simulink model "DNNCells_tSPMeA_BatteryPack_Passive100cellBal_RestCycler"  (R2024a)
settings: Solver=VariableStepAuto  StartTime=0.0  StopTime=1E7  RelTol=1e-3
undefined symbols (not defined in the file or in its folder): battery_builder_rtmsupport, gcbh
libraries: fl_lib x38, nesl_utility x36, simulink x26, BatteryLibrary_lib x6
(part 1 of 2)
settings Model: LastModifiedBy=Carlos

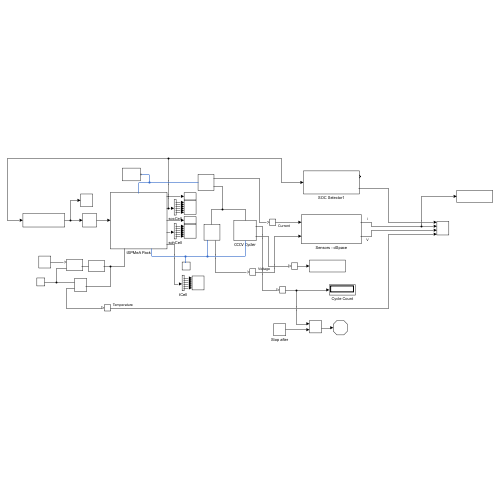
[thumbnail: Simulink's stored preview of the top-level diagram]
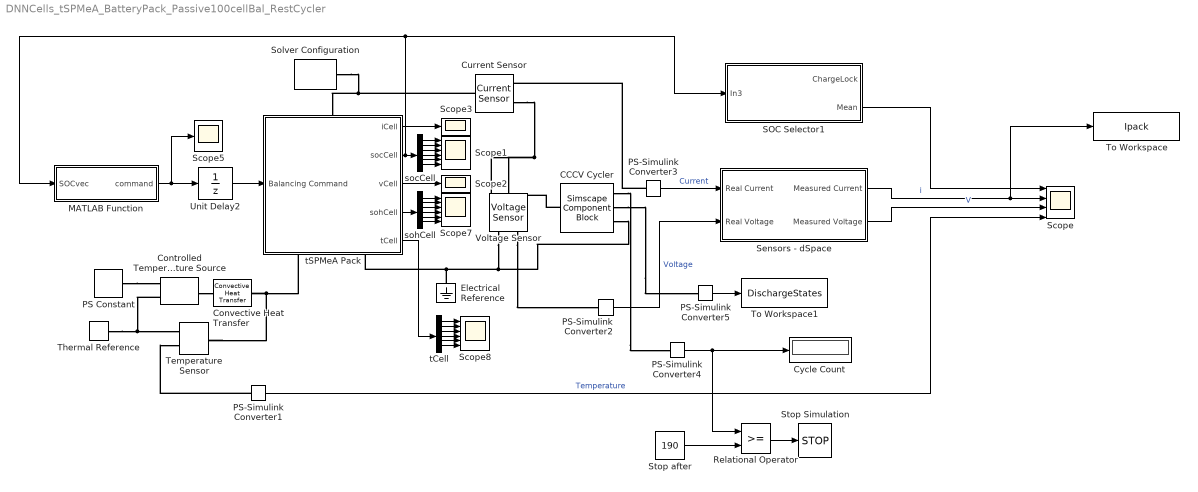
== system DNNCells_tSPMeA_BatteryPack_Passive100cellBal_RestCycler ==
  CCCV Cycler : SimscapeComponentBlock  SourceFile=BatteryCycler_CCCV_DischargeInd  ComponentPath=BatteryCycler_CCCV_DischargeInd  ComponentVariants="[\"BatteryCycler_CCCV_DischargeInd\"]"  ComponentVariantNames="[\"BatteryCycler_CCCV_DischargeInd\"]"  ClassName=BatteryCycler_CCCV_DischargeInd  SchemaVersion=1  Vmax=12.2 V  Vmin=minV V  Ic=iValueC A  Ico=0.25*3 A  Id=iValueD A  tRestC=0 s  tRestD=0 s
      settings: CopyFcn=simscape.engine.sli.internal.componentblockcallback(gcbh,'COPY')  PreCopyFcn=simscape.engine.sli.internal.componentblockcallback(gcbh,'PRECOPY')  PreDeleteFcn=simscape.engine.sli.internal.componentblockcallback(gcbh,'PREDELETE')  InternalSimscapePortConfiguration="{\"Bottom\":[{\"id\":\"n\",\"label\":\"-\",\"type\":\"foundation.electrical.electrical\"}],\"Left\":[],\"Right\":[{\"id\":\"numCyc\",\"label\":\"Cyc#\",\"type\":\"output\"},{\"id\":\"DischargeON\",\"label\":\"dON\",\"type\":\"output\"}],\"Top\":[{\"id\":\"p\",\"label\":\"+\",\"type\":\"foundation.electrical.electrical\"}]}"
      mask Type: A simple battery cycler
      mask Display: color('red');plot([0 1 1 0 0],[0 0 1 1 0]);plot([0.7,1],[1,0.7]);plot(-2,-1.75);plot(3, 1);disp('\n.ssc\nUnresolved')
  Controlled Temperature Source : fl_lib/Thermal/Thermal Sources/Controlled Temperature Source
  Convective Heat Transfer : fl_lib/Thermal/Thermal Elements/Convective Heat Transfer  thermal_type=foundation.enum.constant_variable.constant  area=0.1019 m^2  heat_tr_coeff=5 W/(K*m^2)  min_heat_tr_coeff=1e-3 W/(K*m^2)  T_specify=off  T_priority=None  T=0 K  T_nominal_specify=off  T_nominal_value=1  T_nominal_unit=K  Q_specify=off  Q_priority=None  Q=0 W  Q_nominal_specify=off  Q_nominal_value=1  Q_nominal_unit=W
  Current Sensor : fl_lib/Electrical/Electrical Sensors/Current Sensor
  Cycle Count : Display
  Electrical Reference : fl_lib/Electrical/Electrical Elements/Electrical Reference
  MATLAB Function : MATLAB Function  TreatAsAtomicUnit=on
  PS Constant : fl_lib/Physical Signals/Sources/PS Constant  constant=Rtemp K
  PS-Simulink Converter{1..5} (5 alike) : nesl_utility/PS-Simulink Converter  PhysicalDomain=network_engine_domain  SubClassName=ps_output  LeftPortType=input  RightPortType=output  PseudoPeriodic=off  Frequencies=[]  VectorFormat=inherit  Unit=inherit  AffineConversion=off
  Relational Operator : RelationalOperator  OutDataTypeStr=boolean  RndMeth=Simplest  InputSameDT=off
  SOC Selector1 : Subsystem
  Scope : Scope  NumInputPorts=4
  Scope1 : Scope  NumInputPorts=6
  Scope2 : Scope
  Scope3 : Scope
  Scope5 : Scope
  Scope7 : Scope  NumInputPorts=6
  Scope8 : Scope  NumInputPorts=6
  Sensors - dSpace : Subsystem
  Solver Configuration : nesl_utility/Solver Configuration  PhysicalDomain=network_engine_domain  SubClassName=solver  LeftPortType=input  RightPortType=generic  Tones=[]  Harmonics=[]  SimulateNoise=off  Profile=off  UseLocalSampling=off  EnableSwitchedLinearOptims=on  FrequencyDomain=off  UseCCode=off  RelTol=0.001  AbsTol=0.001  MinStep=1e-09  ToWorkspace=off  RevertToSquareIcSolve=off  NumHomotopyIterations=100  PhasorMode=off  PhasorModeNumHarmonics=1  ConsistencySolver=NEWTON_XTOL_AFTER_FTOL  IndexReductionMethod=DerivativeReplacement  DoDC=off  ResidualTolerance=1e-09  ConsistencyTolSource=GLOBAL  ConsistencyAbsTol=0.001  ConsistencyRelTol=0.001  ConsistencyTolFactor=0.001  UseLocalSolver=off  LocalSolverChoice=NE_BACKWARD_EULER_ADVANCER  ResolveIndetEquations=on  FunctionEvalNumThread=1  LocalSolverSampleTime=0.001  DoFixedCost=off  MaxNonlinIter=3  MaxModeIter=2  ComputeImpulses=off  ImpulseIterations=2  LinearAlgebra=auto  LinearAlgebraNumThread=0  EquationFormulation=NE_TIME_EF  DelaysMemoryBudget=1024  AutomaticFiltering=on  FilteringTimeConstant=0.001  PartitionStorageMethod=AS_NEEDED  PartitionMemoryBudget=1024  PartitionMethod=ROBUST  MultibodyUseLocalSolver=off  MultibodyLocalSolverChoice=ODE1  MultibodyLocalSolverSampleTime=0.001
  Stop Simulation : Stop
  Stop after : Constant  Value=190
  Temperature Sensor : fl_lib/Thermal/Thermal Sensors/Temperature Sensor  temperature_measure=foundation.enum.MeasurementReference.difference
  Thermal Reference : fl_lib/Thermal/Thermal Elements/Thermal Reference
  To Workspace : ToWorkspace  VariableName=Ipack  SampleTime=-1
  To Workspace1 : ToWorkspace  VariableName=DischargeStates  SampleTime=-1
  Unit Delay2 : UnitDelay  SampleTime=-1  HasFrameUpgradeWarning=on
  Voltage Sensor : fl_lib/Electrical/Electrical Sensors/Voltage Sensor
  socCell : Demux  Outputs=6
  sohCell : Demux  Outputs=6
  tCell : Demux  Outputs=6
  tSPMeA Pack : Subsystem  LoadFcn=battery_builder_rtmsupport('loadfcn',gcbh);
      settings: CopyFcn=battery_builder_rtmsupport('copyfcn',gcbh);  PreCopyFcn=battery_builder_rtmsupport('precopyfcn',gcbh);  PreDeleteFcn=battery_builder_rtmsupport('predeletefcn',gcbh);  PortSchema="{\"entries\":[{\"content\":{\"sides\":[{\"content\":{\"connectorIds\":[\"LConn1\"]},\"type\":\"ConnectorPlacement.EquallySpacedRectSide\",\"uuid\":\"edb5d46f-daf4-45ed-b1d9-08af295e59c6\"},{\"content\":{\"connectorIds\":[\"RConn1\",\"RConn2\"],\"side\":\"RIGHT\"},\"type\":\"ConnectorPlacement.EquallySpacedRectSide\",\"uuid\":\"7cebd990-2869-4bd2-9528-842d68f5845c\"},{\"content\":{\"connectorIds\":[\"In1\"],\"side\":\"TOP\"},\"type\":\"ConnectorPlacement.EquallySpacedRectSide\",\"uuid\":\"ba73c8cc-44ad-460a-9725-00030624eda5\"},{\"content\":{\"connectorIds\":[\"Out1\",\"Out2\",\"Out3\",\"Out4\",\"Out5\"],\"side\":\"BOTTOM\"},\"type\":\"ConnectorPlacement.EquallySpacedRectSide\",\"uuid\":\"cf00b7fe-9012-41be-869c-9f0653cf4178\"}]},\"type\":\"ConnectorPlacement.EquallySpacedConnector\",\"uuid\":\"85879143-d5a0-4157-9373-c0baeacbbffb\"}],\"packageUris\":[\"http://schema.mathworks.com/mf0/Connector/R2020b\"],\"version\":\"1.0\"}"
      mask Display: image('$imagefile')
  wires:
  tSPMeA Pack/2(socCell) -> socCell/1, MATLAB Function/1(SOCvec), SOC Selector1/1(In3)
  PS-Simulink Converter1/1 -> Scope/4  "Temperature"
  tSPMeA Pack/1(iCell) -> Scope3/1
  socCell/1 -> Scope1/1
  PS-Simulink Converter2/1 -> Sensors - dSpace/2(Real Voltage)  "Voltage"
  Sensors - dSpace/1(Measured Current) -> To Workspace/1, Scope/2  "i"
  Sensors - dSpace/2(Measured Voltage) -> Scope/3  "V"
  socCell/2 -> Scope1/2
  socCell/3 -> Scope1/3
  socCell/4 -> Scope1/4
  socCell/5 -> Scope1/5
  socCell/6 -> Scope1/6
  Unit Delay2/1 -> tSPMeA Pack/1(Balancing Command)
  tSPMeA Pack/3(vCell) -> Scope2/1
  MATLAB Function/1(command) -> Scope5/1, Unit Delay2/1
  tSPMeA Pack/4(sohCell) -> sohCell/1
  sohCell/1 -> Scope7/1
  sohCell/2 -> Scope7/2
  sohCell/3 -> Scope7/3
  sohCell/4 -> Scope7/4
  sohCell/5 -> Scope7/5
  sohCell/6 -> Scope7/6
  tCell/5 -> Scope8/5
  tCell/1 -> Scope8/1
  tCell/6 -> Scope8/6
  tCell/4 -> Scope8/4
  tCell/3 -> Scope8/3
  tCell/2 -> Scope8/2
  tSPMeA Pack/5(tCell) -> tCell/1
  PS-Simulink Converter3/1 -> Sensors - dSpace/1(Real Current)  "Current"
  SOC Selector1/2(Mean) -> Scope/1
  PS-Simulink Converter4/1 -> Relational Operator/1, Cycle Count/1
  Relational Operator/1 -> Stop Simulation/1
  Stop after/1 -> Relational Operator/2
  PS-Simulink Converter5/1 -> To Workspace1/1
  connections:
  Voltage Sensor/RConn2 -- CCCV Cycler/RConn3 -- Electrical Reference/LConn1 -- tSPMeA Pack/RConn2
  Solver Configuration/RConn1 -- tSPMeA Pack/LConn1 -- Current Sensor/LConn1
  Convective Heat Transfer/LConn1 -- tSPMeA Pack/RConn1 -- Temperature Sensor/LConn1
  Controlled Temperature Source/RConn2 -- Temperature Sensor/RConn1 -- Thermal Reference/LConn1
  PS Constant/RConn1 -- Controlled Temperature Source/RConn1
  Voltage Sensor/RConn1 -- PS-Simulink Converter2/LConn1
  PS-Simulink Converter1/LConn1 -- Temperature Sensor/RConn2
  Controlled Temperature Source/LConn1 -- Convective Heat Transfer/RConn1
  Current Sensor/RConn2 -- CCCV Cycler/LConn1 -- Voltage Sensor/LConn1
  PS-Simulink Converter3/LConn1 -- Current Sensor/RConn1
  CCCV Cycler/RConn1 -- PS-Simulink Converter4/LConn1
  CCCV Cycler/RConn2 -- PS-Simulink Converter5/LConn1

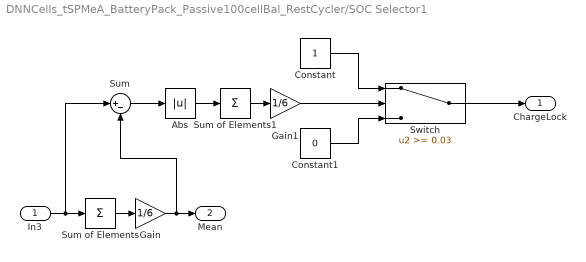
== system DNNCells_tSPMeA_BatteryPack_Passive100cellBal_RestCycler/SOC Selector1 ==
  In3 : Inport
  Abs : Abs  ZeroCross=off  SaturateOnIntegerOverflow=off
  Constant : Constant
  Constant1 : Constant  Value=0
  Gain : Gain  Gain=1/6
  Gain1 : Gain  Gain=1/6
  Sum : Sum  Inputs=|+-
  Sum of Elements : Sum  Inputs=+
  Sum of Elements1 : Sum  Inputs=+
  Switch : Switch  Threshold=0.03  SaturateOnIntegerOverflow=off  InputSameDT=off
  ChargeLock : Outport
  Mean : Outport  Port=2
  wires:
  Gain1/1 -> Switch/2
  In3/1 -> Sum/1, Sum of Elements/1
  Switch/1 -> ChargeLock/1
  Sum of Elements/1 -> Gain/1
  Gain/1 -> Mean/1, Sum/2
  Sum/1 -> Abs/1
  Sum of Elements1/1 -> Gain1/1
  Abs/1 -> Sum of Elements1/1
  Constant/1 -> Switch/1
  Constant1/1 -> Switch/3

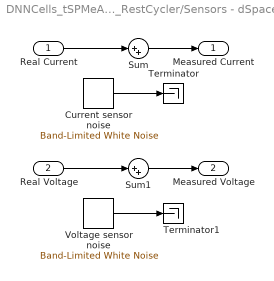
== system DNNCells_tSPMeA_BatteryPack_Passive100cellBal_RestCycler/Sensors - dSpace ==
  Real Current : Inport
  Real Voltage : Inport  Port=2
  Current sensor noise : simulink/Sources/Band-Limited White Noise  Cov=1e-3  Ts=1  seed=1
  Sum : Sum  Inputs=|++
  Sum1 : Sum  Inputs=|++
  Terminator : Terminator
  Terminator1 : Terminator
  Voltage sensor noise : simulink/Sources/Band-Limited White Noise  Cov=1e-3  Ts=1  seed=23341
  Measured Current : Outport
  Measured Voltage : Outport  Port=2
  wires:
  Voltage sensor noise/1 -> Terminator1/1
  Current sensor noise/1 -> Terminator/1
  Real Current/1 -> Sum/1
  Sum1/1 -> Measured Voltage/1
  Sum/1 -> Measured Current/1
  Real Voltage/1 -> Sum1/1

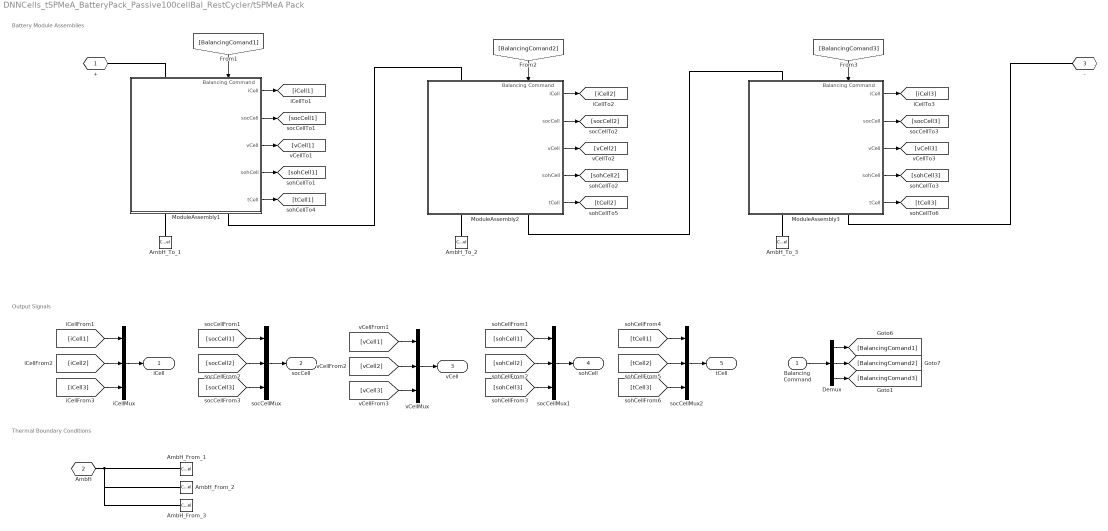
== system DNNCells_tSPMeA_BatteryPack_Passive100cellBal_RestCycler/tSPMeA Pack ==
  note: Thermal Boundary Conditions
  note: Output Signals
  note: Battery Module Assemblies
  Balancing Command : Inport
  AmbH_From_1 : ConnectionLabel  Label=ambH_1
  AmbH_From_2 : ConnectionLabel  Label=ambH_2
  AmbH_From_3 : ConnectionLabel  Label=ambH_3
  AmbH_To_1 : ConnectionLabel  Label=ambH_1
  AmbH_To_2 : ConnectionLabel  Label=ambH_2
  AmbH_To_3 : ConnectionLabel  Label=ambH_3
  Demux : Demux  Outputs=3
  ModuleAssembly1 : Subsystem  LoadFcn=battery_builder_rtmsupport('loadfcn',gcbh);
      settings: CopyFcn=battery_builder_rtmsupport('copyfcn',gcbh);  PreCopyFcn=battery_builder_rtmsupport('precopyfcn',gcbh);  PreDeleteFcn=battery_builder_rtmsupport('predeletefcn',gcbh);  PortSchema="{\"entries\":[{\"content\":{\"sides\":[{\"content\":{\"connectorIds\":[\"LConn1\",\"In1\"]},\"type\":\"ConnectorPlacement.EquallySpacedRectSide\",\"uuid\":\"edb5d46f-daf4-45ed-b1d9-08af295e59c6\"},{\"content\":{\"connectorIds\":[\"RConn1\",\"RConn2\"],\"side\":\"RIGHT\"},\"type\":\"ConnectorPlacement.EquallySpacedRectSide\",\"uuid\":\"7cebd990-2869-4bd2-9528-842d68f5845c\"},{\"content\":{\"side\":\"TOP\"},\"type\":\"ConnectorPlacement.EquallySpacedRectSide\",\"uuid\":\"ba73c8cc-44ad-460a-9725-00030624eda5\"},{\"content\":{\"connectorIds\":[\"Out1\",\"Out2\",\"Out3\",\"Out4\",\"Out5\"],\"side\":\"BOTTOM\"},\"type\":\"ConnectorPlacement.EquallySpacedRectSide\",\"uuid\":\"b96a0b88-50ee-41bf-8d2d-c67f3b56e673\"}]},\"type\":\"ConnectorPlacement.EquallySpacedConnector\",\"uuid\":\"85879143-d5a0-4157-9373-c0baeacbbffb\"}],\"packageUris\":[\"http://schema.mathworks.com/mf0/Connector/R2020b\"],\"version\":\"1.0\"}"
      mask Display: image('$imagefile')
  ModuleAssembly2 : Subsystem  LoadFcn=battery_builder_rtmsupport('loadfcn',gcbh);
      settings: CopyFcn=battery_builder_rtmsupport('copyfcn',gcbh);  PreCopyFcn=battery_builder_rtmsupport('precopyfcn',gcbh);  PreDeleteFcn=battery_builder_rtmsupport('predeletefcn',gcbh);  PortSchema="{\"entries\":[{\"content\":{\"sides\":[{\"content\":{\"connectorIds\":[\"LConn1\",\"In1\"]},\"type\":\"ConnectorPlacement.EquallySpacedRectSide\",\"uuid\":\"dd7ab120-3122-47d6-b9c0-1a2825ecd0ca\"},{\"content\":{\"connectorIds\":[\"RConn1\",\"RConn2\"],\"side\":\"RIGHT\"},\"type\":\"ConnectorPlacement.EquallySpacedRectSide\",\"uuid\":\"13815264-ae91-489b-9e13-d335b01da95f\"},{\"content\":{\"side\":\"TOP\"},\"type\":\"ConnectorPlacement.EquallySpacedRectSide\",\"uuid\":\"875c934a-9cf0-4e5f-925c-8403af159523\"},{\"content\":{\"connectorIds\":[\"Out1\",\"Out2\",\"Out3\",\"Out4\",\"Out5\"],\"side\":\"BOTTOM\"},\"type\":\"ConnectorPlacement.EquallySpacedRectSide\",\"uuid\":\"df07df11-67db-4158-b82e-6d351e2aa647\"}]},\"type\":\"ConnectorPlacement.EquallySpacedConnector\",\"uuid\":\"be5d6b1a-4c3a-4498-bd25-1386c1c651b9\"}],\"packageUris\":[\"http://schema.mathworks.com/mf0/Connector/R2020b\"],\"version\":\"1.0\"}"
      mask Display: image('$imagefile')
  ModuleAssembly3 : Subsystem  LoadFcn=battery_builder_rtmsupport('loadfcn',gcbh);
      settings: CopyFcn=battery_builder_rtmsupport('copyfcn',gcbh);  PreCopyFcn=battery_builder_rtmsupport('precopyfcn',gcbh);  PreDeleteFcn=battery_builder_rtmsupport('predeletefcn',gcbh);  PortSchema="{\"entries\":[{\"content\":{\"sides\":[{\"content\":{\"connectorIds\":[\"LConn1\",\"In1\"]},\"type\":\"ConnectorPlacement.EquallySpacedRectSide\",\"uuid\":\"dd7ab120-3122-47d6-b9c0-1a2825ecd0ca\"},{\"content\":{\"connectorIds\":[\"RConn1\",\"RConn2\"],\"side\":\"RIGHT\"},\"type\":\"ConnectorPlacement.EquallySpacedRectSide\",\"uuid\":\"13815264-ae91-489b-9e13-d335b01da95f\"},{\"content\":{\"side\":\"TOP\"},\"type\":\"ConnectorPlacement.EquallySpacedRectSide\",\"uuid\":\"875c934a-9cf0-4e5f-925c-8403af159523\"},{\"content\":{\"connectorIds\":[\"Out1\",\"Out2\",\"Out3\",\"Out4\",\"Out5\"],\"side\":\"BOTTOM\"},\"type\":\"ConnectorPlacement.EquallySpacedRectSide\",\"uuid\":\"995c3d86-7d4c-433a-9b72-f906efb5e596\"}]},\"type\":\"ConnectorPlacement.EquallySpacedConnector\",\"uuid\":\"be5d6b1a-4c3a-4498-bd25-1386c1c651b9\"}],\"packageUris\":[\"http://schema.mathworks.com/mf0/Connector/R2020b\"],\"version\":\"1.0\"}"
      mask Display: image('$imagefile')
  iCellMux : Mux  Inputs=3
  socCellMux : Mux  Inputs=3
  socCellMux1 : Mux  Inputs=3
  socCellMux2 : Mux  Inputs=3
  vCellMux : Mux  Inputs=3
  + : PMIOPort  Side=Left
  AmbH : PMIOPort  Port=2  Side=Right  ConnectionType=Connection: foundation.thermal.thermal
  - : PMIOPort  Port=3  Side=Right
  iCell : Outport
  socCell : Outport  Port=2
  vCell : Outport  Port=3
  sohCell : Outport  Port=4
  tCell : Outport  Port=5
  wires:
  ModuleAssembly2/3(vCell) -> [vCell2]
  ModuleAssembly2/2(socCell) -> [socCell2]
  ModuleAssembly2/1(iCell) -> [iCell2]
  ModuleAssembly1/3(vCell) -> [vCell1]
  ModuleAssembly1/2(socCell) -> [socCell1]
  ModuleAssembly1/1(iCell) -> [iCell1]
  iCellMux/1 -> iCell/1
  [iCell3] -> iCellMux/3
  [iCell1] -> iCellMux/1
  [iCell2] -> iCellMux/2
  [socCell1] -> socCellMux/1
  [socCell2] -> socCellMux/2
  [socCell3] -> socCellMux/3
  socCellMux/1 -> socCell/1
  [vCell2] -> vCellMux/2
  vCellMux/1 -> vCell/1
  [vCell1] -> vCellMux/1
  [vCell3] -> vCellMux/3
  ModuleAssembly3/2(socCell) -> [socCell3]
  ModuleAssembly3/3(vCell) -> [vCell3]
  ModuleAssembly3/1(iCell) -> [iCell3]
  [BalancingComand1] -> ModuleAssembly1/1(Balancing Command)
  [BalancingComand2] -> ModuleAssembly2/1(Balancing Command)
  [BalancingComand3] -> ModuleAssembly3/1(Balancing Command)
  Balancing Command/1 -> Demux/1
  Demux/1 -> [BalancingComand1]
  Demux/2 -> [BalancingComand2]
  Demux/3 -> [BalancingComand3]
  ModuleAssembly1/4(sohCell) -> [sohCell1]
  [sohCell3] -> socCellMux1/3
  socCellMux1/1 -> sohCell/1
  [sohCell2] -> socCellMux1/2
  [sohCell1] -> socCellMux1/1
  ModuleAssembly2/4(sohCell) -> [sohCell2]
  ModuleAssembly3/4(sohCell) -> [sohCell3]
  [tCell1] -> socCellMux2/1
  [tCell2] -> socCellMux2/2
  [tCell3] -> socCellMux2/3
  socCellMux2/1 -> tCell/1
  ModuleAssembly1/5(tCell) -> [tCell1]
  ModuleAssembly2/5(tCell) -> [tCell2]
  ModuleAssembly3/5(tCell) -> [tCell3]
  connections:
  ModuleAssembly2/RConn1 -- AmbH_To_2/LConn1
  AmbH_From_1/LConn1 -- AmbH/RConn1 -- AmbH_From_2/LConn1 -- AmbH_From_3/LConn1
  AmbH_To_1/LConn1 -- ModuleAssembly1/RConn1
  -/RConn1 -- ModuleAssembly3/RConn2
  ModuleAssembly1/LConn1 -- +/RConn1
  ModuleAssembly2/LConn1 -- ModuleAssembly1/RConn2
  ModuleAssembly3/RConn1 -- AmbH_To_3/LConn1
  ModuleAssembly2/RConn2 -- ModuleAssembly3/LConn1

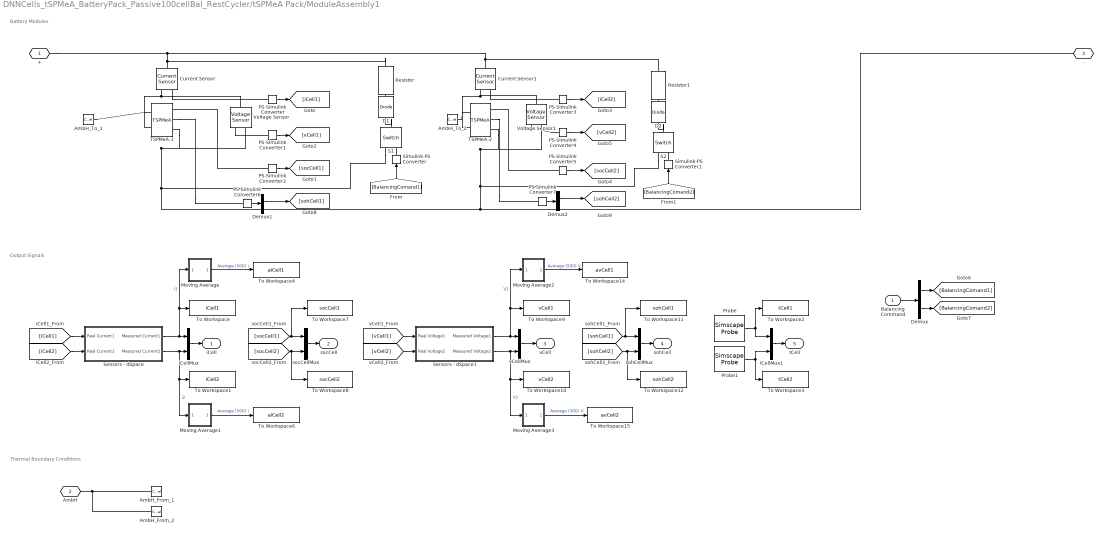
== system DNNCells_tSPMeA_BatteryPack_Passive100cellBal_RestCycler/tSPMeA Pack/ModuleAssembly1 ==
  note: Battery Modules
  note: Output Signals
  note: Thermal Boundary Conditions
  Balancing Command : Inport
  AmbH_From_1 : ConnectionLabel  Label=ambH_1
  AmbH_From_2 : ConnectionLabel  Label=ambH_2
  AmbH_To_1 : ConnectionLabel  Label=ambH_1
  AmbH_To_2 : ConnectionLabel  Label=ambH_2
  Current Sensor : fl_lib/Electrical/Electrical Sensors/Current Sensor
  Current Sensor1 : fl_lib/Electrical/Electrical Sensors/Current Sensor
  D1 : fl_lib/Electrical/Electrical Elements/Diode  Vf=0.6 V  Ron=0.3 Ohm  Goff=1e-8 1/Ohm  i_specify=off  i_priority=None  i=0 A  i_nominal_specify=off  i_nominal_value=1  i_nominal_unit=A  v_specify=off  v_priority=None  v=0 V  v_nominal_specify=off  v_nominal_value=1  v_nominal_unit=V
      settings: LogSimulationData=on
  D2 : fl_lib/Electrical/Electrical Elements/Diode  Vf=0.6 V  Ron=0.3 Ohm  Goff=1e-8 1/Ohm  i_specify=off  i_priority=None  i=0 A  i_nominal_specify=off  i_nominal_value=1  i_nominal_unit=A  v_specify=off  v_priority=None  v=0 V  v_nominal_specify=off  v_nominal_value=1  v_nominal_unit=V
      settings: LogSimulationData=on
  Demux : Demux  Outputs=2
  Demux1 : Demux
  Demux2 : Demux
  Moving Average : Subsystem
  Moving Average1 : Subsystem
  Moving Average2 : Subsystem
  Moving Average3 : Subsystem
  PS-Simulink Converter{,1..7} (8 alike) : nesl_utility/PS-Simulink Converter  PhysicalDomain=network_engine_domain  SubClassName=ps_output  LeftPortType=input  RightPortType=output  PseudoPeriodic=off  Frequencies=[]  VectorFormat=inherit  Unit=inherit  AffineConversion=off
  Probe : SimscapeProbe  BoundBlock=211  Variables={T}
  Probe1 : SimscapeProbe  BoundBlock=212  Variables={T}
  Resistor : fl_lib/Electrical/Electrical Elements/Resistor  R=0.001 Ohm  i_specify=off  i_priority=None  i=0 A  i_nominal_specify=off  i_nominal_value=1  i_nominal_unit=A  v_specify=off  v_priority=None  v=0 V  v_nominal_specify=off  v_nominal_value=1  v_nominal_unit=V
  Resistor1 : fl_lib/Electrical/Electrical Elements/Resistor  R=0.001 Ohm  i_specify=off  i_priority=None  i=0 A  i_nominal_specify=off  i_nominal_value=1  i_nominal_unit=A  v_specify=off  v_priority=None  v=0 V  v_nominal_specify=off  v_nominal_value=1  v_nominal_unit=V
  S1 : fl_lib/Electrical/Electrical Elements/Switch  R_closed=0.01 Ohm  G_open=1e-8 1/Ohm  Threshold=0.5  i_specify=off  i_priority=None  i=0 A  i_nominal_specify=off  i_nominal_value=1  i_nominal_unit=A  v_specify=off  v_priority=None  v=0 V  v_nominal_specify=off  v_nominal_value=1  v_nominal_unit=V
  S2 : fl_lib/Electrical/Electrical Elements/Switch  R_closed=0.01 Ohm  G_open=1e-8 1/Ohm  Threshold=0.5  i_specify=off  i_priority=None  i=0 A  i_nominal_specify=off  i_nominal_value=1  i_nominal_unit=A  v_specify=off  v_priority=None  v=0 V  v_nominal_specify=off  v_nominal_value=1  v_nominal_unit=V
  Sensors - dSpace : Subsystem
  Sensors - dSpace1 : Subsystem
  Simulink-PS Converter : nesl_utility/Simulink-PS Converter  PhysicalDomain=network_engine_domain  SubClassName=ps_input  LeftPortType=input  RightPortType=output  PseudoPeriodic=off  Frequencies=[]  NoiseDistribution=none  NoiseParameters=[]  Unit=1  AffineConversion=off  FilteringAndDerivatives=provide  SimscapeFilterOrder=1  InputFilterTimeConstant=0.001  UdotUserProvided=0
  Simulink-PS Converter1 : nesl_utility/Simulink-PS Converter  PhysicalDomain=network_engine_domain  SubClassName=ps_input  LeftPortType=input  RightPortType=output  PseudoPeriodic=off  Frequencies=[]  NoiseDistribution=none  NoiseParameters=[]  Unit=1  AffineConversion=off  FilteringAndDerivatives=provide  SimscapeFilterOrder=1  InputFilterTimeConstant=0.001  UdotUserProvided=0
  TSPMeA-1 : BatteryLibrary_lib/Models/TSPMeA  z0=cSoc1  T0=Ctemp1 K  eps_n0=0.25  Lf0=5E-3 um  Cn=4.9 A*hr  DnRef=3.3E-14 m^2/s  DpRef=4E-15 m^2/s  sigma_nRef=215 S/m  sigma_eRef=1.2 S/m  sigma_pRef=0.18 S/m  tr=0.2594  ce0=1000 mol/m^3  cn_max=33133 mol/m^3  cp_max=63104 mol/m^3  sn_max=0.9014  sn_min=0.0279  sp_max=0.9072  sp_min=0.2567  knRef=6.48E-7 A*m^(5/2)/mol^(3/2)  kpRef=3.42E-6 A*m^(5/2)/mol^(3/2)  Cp=110 J/K  Tref=298 K  Ea_kn=1 kJ/mol  Ea_kp=1 kJ/mol  Ea_Dn=75 kJ/mol  Ea_De=1.2 kJ/mol  Ea_Dp=10 kJ/mol  Ea_sigman=80 kJ/mol  Ea_sigmae=80 kJ/mol  Ea_sigmap=80 kJ/mol  Ea_ksei=1 kJ/mol  Ea_Dsei=1 kJ/mol  Ea_sigmasei=1 kJ/mol  Ea_kLi=1 kJ/mol  kseiRef=1E-12 m/s  DseiRef=2E-19 m^2/s  sigma_seiRef=5E-6 S/m  Msei=0.162 kg/mol  pho_sei=1690 kg/m^3  Usei=0 V  csei0=4541 mol/m^3  kLiRef=1E-11 m/s  ULi=0 V  MLi=6.94E-3 kg/mol  pho_Li=534 kg/m^3  Ln=85.2 um  Ls=12 um  Lp=75.6 um  Area_p=1027 cm^2  eps_s=0.47  eps_p=0.335  Rn=5.86 um  Rp=5.22 um  an=3.84E5 1/m  ap=3.82E5 1/m
      settings: LogSimulationData=on  InternalSimscapePortConfiguration="{\"Bottom\":[{\"id\":\"n\",\"label\":\"-\",\"type\":\"foundation.electrical.electrical\"}],\"Left\":[{\"id\":\"Hi\",\"label\":\"H\",\"type\":\"foundation.thermal.thermal\"}],\"Right\":[{\"id\":\"z\",\"label\":\"SoC\",\"type\":\"output\"},{\"id\":\"Lf_bar\",\"label\":\"sohF\",\"type\":\"output\"},{\"id\":\"SoH_Cn\",\"label\":\"sohC\",\"type\":\"output\"},{\"id\":\"pots\",\"label\":\"Pots\",\"type\":\"output\"}],\"Top\":[{\"id\":\"p\",\"label\":\"+\",\"type\":\"foundation.electrical.electrical\"}]}"
  TSPMeA-2 : BatteryLibrary_lib/Models/TSPMeA  z0=cSoc2  T0=Ctemp2 K  eps_n0=0.25  Lf0=5E-3 um  Cn=4.9 A*hr  DnRef=3.3E-14 m^2/s  DpRef=4E-15 m^2/s  sigma_nRef=215 S/m  sigma_eRef=1.2 S/m  sigma_pRef=0.18 S/m  tr=0.2594  ce0=1000 mol/m^3  cn_max=33133 mol/m^3  cp_max=63104 mol/m^3  sn_max=0.9014  sn_min=0.0279  sp_max=0.9072  sp_min=0.2567  knRef=6.48E-7 A*m^(5/2)/mol^(3/2)  kpRef=3.42E-6 A*m^(5/2)/mol^(3/2)  Cp=110 J/K  Tref=298 K  Ea_kn=1 kJ/mol  Ea_kp=1 kJ/mol  Ea_Dn=75 kJ/mol  Ea_De=1.2 kJ/mol  Ea_Dp=10 kJ/mol  Ea_sigman=80 kJ/mol  Ea_sigmae=80 kJ/mol  Ea_sigmap=80 kJ/mol  Ea_ksei=1 kJ/mol  Ea_Dsei=1 kJ/mol  Ea_sigmasei=1 kJ/mol  Ea_kLi=1 kJ/mol  kseiRef=1E-12 m/s  DseiRef=2E-19 m^2/s  sigma_seiRef=5E-6 S/m  Msei=0.162 kg/mol  pho_sei=1690 kg/m^3  Usei=0 V  csei0=4541 mol/m^3  kLiRef=1E-11 m/s  ULi=0 V  MLi=6.94E-3 kg/mol  pho_Li=534 kg/m^3  Ln=85.2 um  Ls=12 um  Lp=75.6 um  Area_p=1027 cm^2  eps_s=0.47  eps_p=0.335  Rn=5.86 um  Rp=5.22 um  an=3.84E5 1/m  ap=3.82E5 1/m
      settings: InternalSimscapePortConfiguration="{\"Bottom\":[{\"id\":\"n\",\"label\":\"-\",\"type\":\"foundation.electrical.electrical\"}],\"Left\":[{\"id\":\"Hi\",\"label\":\"H\",\"type\":\"foundation.thermal.thermal\"}],\"Right\":[{\"id\":\"z\",\"label\":\"SoC\",\"type\":\"output\"},{\"id\":\"Lf_bar\",\"label\":\"sohF\",\"type\":\"output\"},{\"id\":\"SoH_Cn\",\"label\":\"sohC\",\"type\":\"output\"},{\"id\":\"pots\",\"label\":\"Pots\",\"type\":\"output\"}],\"Top\":[{\"id\":\"p\",\"label\":\"+\",\"type\":\"foundation.electrical.electrical\"}]}"
  To Workspace : ToWorkspace  VariableName=iCell1  SampleTime=-1
  To Workspace1 : ToWorkspace  VariableName=iCell2  SampleTime=-1
  To Workspace10 : ToWorkspace  VariableName=vCell2  SampleTime=-1
  To Workspace11 : ToWorkspace  VariableName=sohCell1  SampleTime=-1
  To Workspace12 : ToWorkspace  VariableName=sohCell2  SampleTime=-1
  To Workspace14 : ToWorkspace  VariableName=avCell1  SampleTime=-1
  To Workspace15 : ToWorkspace  VariableName=avCell2  SampleTime=-1
  To Workspace2 : ToWorkspace  VariableName=tCell1  SampleTime=-1
  To Workspace3 : ToWorkspace  VariableName=tCell2  SampleTime=-1
  To Workspace4 : ToWorkspace  VariableName=aiCell1  SampleTime=-1
  To Workspace6 : ToWorkspace  VariableName=aiCell2  SampleTime=-1
  To Workspace7 : ToWorkspace  VariableName=socCell1  SampleTime=-1
  To Workspace8 : ToWorkspace  VariableName=socCell2  SampleTime=-1
  To Workspace9 : ToWorkspace  VariableName=vCell1  SampleTime=-1
  Voltage Sensor : fl_lib/Electrical/Electrical Sensors/Voltage Sensor
  Voltage Sensor1 : fl_lib/Electrical/Electrical Sensors/Voltage Sensor
  iCellMux : Mux  Inputs=2
  iCellMux1 : Mux  Inputs=2
  socCellMux : Mux  Inputs=2
  sohCellMux : Mux  Inputs=2
  vCellMux : Mux  Inputs=2
  + : PMIOPort  Side=Left
  AmbH : PMIOPort  Port=2  Side=Right  ConnectionType=Connection: foundation.thermal.thermal
  - : PMIOPort  Port=3  Side=Right
  iCell : Outport
  socCell : Outport  Port=2
  vCell : Outport  Port=3
  sohCell : Outport  Port=4
  tCell : Outport  Port=5
  wires:
  PS-Simulink Converter1/1 -> [vCell1]
  PS-Simulink Converter2/1 -> [socCell1]
  PS-Simulink Converter/1 -> [iCell1]
  iCellMux/1 -> iCell/1
  [iCell1] -> Sensors - dSpace/1(Real Current1)
  socCellMux/1 -> socCell/1
  vCellMux/1 -> vCell/1
  PS-Simulink Converter3/1 -> [iCell2]
  PS-Simulink Converter4/1 -> [vCell2]
  PS-Simulink Converter5/1 -> [socCell2]
  Demux/1 -> [BalancingComand1]
  Demux/2 -> [BalancingComand2]
  Balancing Command/1 -> Demux/1
  [BalancingComand1] -> Simulink-PS Converter/1
  [BalancingComand2] -> Simulink-PS Converter1/1
  PS-Simulink Converter6/1 -> Demux1/1
  Demux1/2 -> [sohCell1]
  Demux2/2 -> [sohCell2]
  PS-Simulink Converter7/1 -> Demux2/1
  sohCellMux/1 -> sohCell/1
  [socCell2] -> To Workspace8/1, socCellMux/2
  [socCell1] -> To Workspace7/1, socCellMux/1
  [sohCell2] -> sohCellMux/2, To Workspace12/1
  [sohCell1] -> To Workspace11/1, sohCellMux/1
  iCellMux1/1 -> tCell/1
  Probe/1 -> To Workspace2/1, iCellMux1/1
  Probe1/1 -> To Workspace3/1, iCellMux1/2
  Moving Average/1(Out1) -> To Workspace4/1  "Average (500) i"
  Moving Average1/1(Out1) -> To Workspace6/1  "Average (500) i"
  Moving Average2/1(Out1) -> To Workspace14/1  "Average (500) V"
  Moving Average3/1(Out1) -> To Workspace15/1  "Average (500) V"
  Sensors - dSpace/1(Measured Current1) -> To Workspace/1, Moving Average/1(Measured Current), iCellMux/1  "i1"
  [iCell2] -> Sensors - dSpace/2(Real Current2)
  Sensors - dSpace/2(Measured Current2) -> Moving Average1/1(Measured Voltage), To Workspace1/1, iCellMux/2  "i2"
  [vCell1] -> Sensors - dSpace1/1(Real Voltage1)
  [vCell2] -> Sensors - dSpace1/2(Real Voltage2)
  Sensors - dSpace1/1(Measured Voltage1) -> Moving Average2/1(Measured Current), To Workspace9/1, vCellMux/1  "V1"
  Sensors - dSpace1/2(Measured Voltage2) -> Moving Average3/1(Measured Voltage), To Workspace10/1, vCellMux/2  "V2"
  connections:
  PS-Simulink Converter2/LConn1 -- TSPMeA-1/RConn1
  Voltage Sensor/RConn1 -- PS-Simulink Converter1/LConn1
  Current Sensor/RConn1 -- PS-Simulink Converter/LConn1
  Current Sensor/RConn2 -- TSPMeA-1/LConn2 -- Voltage Sensor/LConn1
  -/RConn1 -- S2/RConn2 -- TSPMeA-2/RConn5 -- Voltage Sensor1/RConn2 -- S1/RConn2 -- TSPMeA-1/RConn5 -- Voltage Sensor/RConn2
  TSPMeA-1/LConn1 -- AmbH_To_1/LConn1
  AmbH/RConn1 -- AmbH_From_1/LConn1 -- AmbH_From_2/LConn1
  +/RConn1 -- Resistor1/LConn1 -- Current Sensor1/LConn1 -- Resistor/LConn1 -- Current Sensor/LConn1
  TSPMeA-2/LConn1 -- AmbH_To_2/LConn1
  Current Sensor1/RConn2 -- Voltage Sensor1/LConn1 -- TSPMeA-2/LConn2
  Current Sensor1/RConn1 -- PS-Simulink Converter3/LConn1
  PS-Simulink Converter5/LConn1 -- TSPMeA-2/RConn1
  PS-Simulink Converter4/LConn1 -- Voltage Sensor1/RConn1
  D1/LConn1 -- Resistor/RConn1
  S1/LConn1 -- D1/RConn1
  Simulink-PS Converter/RConn1 -- S1/RConn1
  Simulink-PS Converter1/RConn1 -- S2/RConn1
  D2/LConn1 -- Resistor1/RConn1
  S2/LConn1 -- D2/RConn1
  TSPMeA-1/RConn3 -- PS-Simulink Converter6/LConn1
  TSPMeA-2/RConn3 -- PS-Simulink Converter7/LConn1

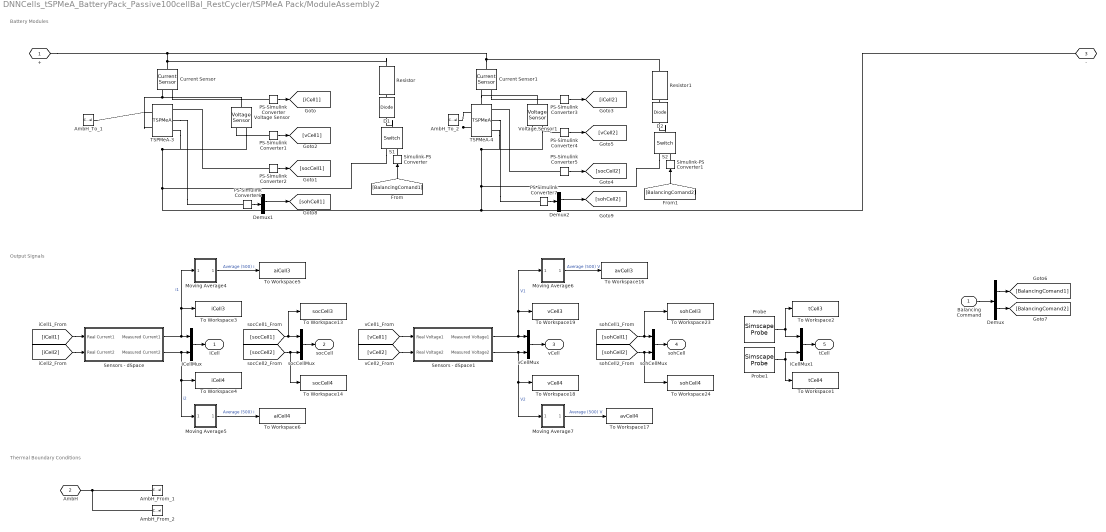
== system DNNCells_tSPMeA_BatteryPack_Passive100cellBal_RestCycler/tSPMeA Pack/ModuleAssembly2 ==
  note: Thermal Boundary Conditions
  note: Battery Modules
  note: Output Signals
  Balancing Command : Inport
  AmbH_From_1 : ConnectionLabel  Label=ambH_1
  AmbH_From_2 : ConnectionLabel  Label=ambH_2
  AmbH_To_1 : ConnectionLabel  Label=ambH_1
  AmbH_To_2 : ConnectionLabel  Label=ambH_2
  Current Sensor : fl_lib/Electrical/Electrical Sensors/Current Sensor
  Current Sensor1 : fl_lib/Electrical/Electrical Sensors/Current Sensor
  D1 : fl_lib/Electrical/Electrical Elements/Diode  Vf=0.6 V  Ron=0.3 Ohm  Goff=1e-8 1/Ohm  i_specify=off  i_priority=None  i=0 A  i_nominal_specify=off  i_nominal_value=1  i_nominal_unit=A  v_specify=off  v_priority=None  v=0 V  v_nominal_specify=off  v_nominal_value=1  v_nominal_unit=V
      settings: LogSimulationData=on
  D2 : fl_lib/Electrical/Electrical Elements/Diode  Vf=0.6 V  Ron=0.3 Ohm  Goff=1e-8 1/Ohm  i_specify=off  i_priority=None  i=0 A  i_nominal_specify=off  i_nominal_value=1  i_nominal_unit=A  v_specify=off  v_priority=None  v=0 V  v_nominal_specify=off  v_nominal_value=1  v_nominal_unit=V
      settings: LogSimulationData=on
  Demux : Demux  Outputs=2
  Demux1 : Demux
  Demux2 : Demux
  Moving Average4 : Subsystem
  Moving Average5 : Subsystem
  Moving Average6 : Subsystem
  Moving Average7 : Subsystem
  PS-Simulink Converter{,1..7} (8 alike) : nesl_utility/PS-Simulink Converter  PhysicalDomain=network_engine_domain  SubClassName=ps_output  LeftPortType=input  RightPortType=output  PseudoPeriodic=off  Frequencies=[]  VectorFormat=inherit  Unit=inherit  AffineConversion=off
  Probe : SimscapeProbe  BoundBlock=374  Variables={T}
  Probe1 : SimscapeProbe  BoundBlock=375  Variables={T}
  Resistor : fl_lib/Electrical/Electrical Elements/Resistor  R=0.001 mOhm  i_specify=off  i_priority=None  i=0 A  i_nominal_specify=off  i_nominal_value=1  i_nominal_unit=A  v_specify=off  v_priority=None  v=0 V  v_nominal_specify=off  v_nominal_value=1  v_nominal_unit=V
  Resistor1 : fl_lib/Electrical/Electrical Elements/Resistor  R=0.001 mOhm  i_specify=off  i_priority=None  i=0 A  i_nominal_specify=off  i_nominal_value=1  i_nominal_unit=A  v_specify=off  v_priority=None  v=0 V  v_nominal_specify=off  v_nominal_value=1  v_nominal_unit=V
  S1 : fl_lib/Electrical/Electrical Elements/Switch  R_closed=0.01 Ohm  G_open=1e-8 1/Ohm  Threshold=0.5  i_specify=off  i_priority=None  i=0 A  i_nominal_specify=off  i_nominal_value=1  i_nominal_unit=A  v_specify=off  v_priority=None  v=0 V  v_nominal_specify=off  v_nominal_value=1  v_nominal_unit=V
  S2 : fl_lib/Electrical/Electrical Elements/Switch  R_closed=0.01 Ohm  G_open=1e-8 1/Ohm  Threshold=0.5  i_specify=off  i_priority=None  i=0 A  i_nominal_specify=off  i_nominal_value=1  i_nominal_unit=A  v_specify=off  v_priority=None  v=0 V  v_nominal_specify=off  v_nominal_value=1  v_nominal_unit=V
  Sensors - dSpace : Subsystem
  Sensors - dSpace1 : Subsystem
  Simulink-PS Converter : nesl_utility/Simulink-PS Converter  PhysicalDomain=network_engine_domain  SubClassName=ps_input  LeftPortType=input  RightPortType=output  PseudoPeriodic=off  Frequencies=[]  NoiseDistribution=none  NoiseParameters=[]  Unit=1  AffineConversion=off  FilteringAndDerivatives=provide  SimscapeFilterOrder=1  InputFilterTimeConstant=0.001  UdotUserProvided=0
  Simulink-PS Converter1 : nesl_utility/Simulink-PS Converter  PhysicalDomain=network_engine_domain  SubClassName=ps_input  LeftPortType=input  RightPortType=output  PseudoPeriodic=off  Frequencies=[]  NoiseDistribution=none  NoiseParameters=[]  Unit=1  AffineConversion=off  FilteringAndDerivatives=provide  SimscapeFilterOrder=1  InputFilterTimeConstant=0.001  UdotUserProvided=0
  TSPMeA-3 : BatteryLibrary_lib/Models/TSPMeA  z0=cSoc3  T0=Ctemp3 K  eps_n0=0.25  Lf0=5E-3 um  Cn=4.9 A*hr  DnRef=3.3E-14 m^2/s  DpRef=4E-15 m^2/s  sigma_nRef=215 S/m  sigma_eRef=1.2 S/m  sigma_pRef=0.18 S/m  tr=0.2594  ce0=1000 mol/m^3  cn_max=33133 mol/m^3  cp_max=63104 mol/m^3  sn_max=0.9014  sn_min=0.0279  sp_max=0.9072  sp_min=0.2567  knRef=6.48E-7 A*m^(5/2)/mol^(3/2)  kpRef=3.42E-6 A*m^(5/2)/mol^(3/2)  Cp=110 J/K  Tref=298 K  Ea_kn=1 kJ/mol  Ea_kp=1 kJ/mol  Ea_Dn=75 kJ/mol  Ea_De=1.2 kJ/mol  Ea_Dp=10 kJ/mol  Ea_sigman=80 kJ/mol  Ea_sigmae=80 kJ/mol  Ea_sigmap=80 kJ/mol  Ea_ksei=1 kJ/mol  Ea_Dsei=1 kJ/mol  Ea_sigmasei=1 kJ/mol  Ea_kLi=1 kJ/mol  kseiRef=1E-12 m/s  DseiRef=2E-19 m^2/s  sigma_seiRef=5E-6 S/m  Msei=0.162 kg/mol  pho_sei=1690 kg/m^3  Usei=0 V  csei0=4541 mol/m^3  kLiRef=1E-11 m/s  ULi=0 V  MLi=6.94E-3 kg/mol  pho_Li=534 kg/m^3  Ln=85.2 um  Ls=12 um  Lp=75.6 um  Area_p=1027 cm^2  eps_s=0.47  eps_p=0.335  Rn=5.86 um  Rp=5.22 um  an=3.84E5 1/m  ap=3.82E5 1/m
      settings: InternalSimscapePortConfiguration="{\"Bottom\":[{\"id\":\"n\",\"label\":\"-\",\"type\":\"foundation.electrical.electrical\"}],\"Left\":[{\"id\":\"Hi\",\"label\":\"H\",\"type\":\"foundation.thermal.thermal\"}],\"Right\":[{\"id\":\"z\",\"label\":\"SoC\",\"type\":\"output\"},{\"id\":\"Lf_bar\",\"label\":\"sohF\",\"type\":\"output\"},{\"id\":\"SoH_Cn\",\"label\":\"sohC\",\"type\":\"output\"},{\"id\":\"pots\",\"label\":\"Pots\",\"type\":\"output\"}],\"Top\":[{\"id\":\"p\",\"label\":\"+\",\"type\":\"foundation.electrical.electrical\"}]}"
  TSPMeA-4 : BatteryLibrary_lib/Models/TSPMeA  z0=cSoc4  T0=Ctemp4 K  eps_n0=0.25  Lf0=5E-3 um  Cn=4.9 A*hr  DnRef=3.3E-14 m^2/s  DpRef=4E-15 m^2/s  sigma_nRef=215 S/m  sigma_eRef=1.2 S/m  sigma_pRef=0.18 S/m  tr=0.2594  ce0=1000 mol/m^3  cn_max=33133 mol/m^3  cp_max=63104 mol/m^3  sn_max=0.9014  sn_min=0.0279  sp_max=0.9072  sp_min=0.2567  knRef=6.48E-7 A*m^(5/2)/mol^(3/2)  kpRef=3.42E-6 A*m^(5/2)/mol^(3/2)  Cp=110 J/K  Tref=298 K  Ea_kn=1 kJ/mol  Ea_kp=1 kJ/mol  Ea_Dn=75 kJ/mol  Ea_De=1.2 kJ/mol  Ea_Dp=10 kJ/mol  Ea_sigman=80 kJ/mol  Ea_sigmae=80 kJ/mol  Ea_sigmap=80 kJ/mol  Ea_ksei=1 kJ/mol  Ea_Dsei=1 kJ/mol  Ea_sigmasei=1 kJ/mol  Ea_kLi=1 kJ/mol  kseiRef=1E-12 m/s  DseiRef=2E-19 m^2/s  sigma_seiRef=5E-6 S/m  Msei=0.162 kg/mol  pho_sei=1690 kg/m^3  Usei=0 V  csei0=4541 mol/m^3  kLiRef=1E-11 m/s  ULi=0 V  MLi=6.94E-3 kg/mol  pho_Li=534 kg/m^3  Ln=85.2 um  Ls=12 um  Lp=75.6 um  Area_p=1027 cm^2  eps_s=0.47  eps_p=0.335  Rn=5.86 um  Rp=5.22 um  an=3.84E5 1/m  ap=3.82E5 1/m
      settings: InternalSimscapePortConfiguration="{\"Bottom\":[{\"id\":\"n\",\"label\":\"-\",\"type\":\"foundation.electrical.electrical\"}],\"Left\":[{\"id\":\"Hi\",\"label\":\"H\",\"type\":\"foundation.thermal.thermal\"}],\"Right\":[{\"id\":\"z\",\"label\":\"SoC\",\"type\":\"output\"},{\"id\":\"Lf_bar\",\"label\":\"sohF\",\"type\":\"output\"},{\"id\":\"SoH_Cn\",\"label\":\"sohC\",\"type\":\"output\"},{\"id\":\"pots\",\"label\":\"Pots\",\"type\":\"output\"}],\"Top\":[{\"id\":\"p\",\"label\":\"+\",\"type\":\"foundation.electrical.electrical\"}]}"
  To Workspace1 : ToWorkspace  VariableName=tCell4  SampleTime=-1
  To Workspace13 : ToWorkspace  VariableName=socCell3  SampleTime=-1
  To Workspace14 : ToWorkspace  VariableName=socCell4  SampleTime=-1
  To Workspace16 : ToWorkspace  VariableName=avCell3  SampleTime=-1
  To Workspace17 : ToWorkspace  VariableName=avCell4  SampleTime=-1
  To Workspace18 : ToWorkspace  VariableName=vCell4  SampleTime=-1
  To Workspace19 : ToWorkspace  VariableName=vCell3  SampleTime=-1
  To Workspace2 : ToWorkspace  VariableName=tCell3  SampleTime=-1
  To Workspace23 : ToWorkspace  VariableName=sohCell3  SampleTime=-1
  To Workspace24 : ToWorkspace  VariableName=sohCell4  SampleTime=-1
  To Workspace3 : ToWorkspace  VariableName=iCell3  SampleTime=-1
  To Workspace4 : ToWorkspace  VariableName=iCell4  SampleTime=-1
  To Workspace5 : ToWorkspace  VariableName=aiCell3  SampleTime=-1
  To Workspace6 : ToWorkspace  VariableName=aiCell4  SampleTime=-1
  Voltage Sensor : fl_lib/Electrical/Electrical Sensors/Voltage Sensor
  Voltage Sensor1 : fl_lib/Electrical/Electrical Sensors/Voltage Sensor
  iCellMux : Mux  Inputs=2
  iCellMux1 : Mux  Inputs=2
  socCellMux : Mux  Inputs=2
  sohCellMux : Mux  Inputs=2
  vCellMux : Mux  Inputs=2
  + : PMIOPort  Side=Left
  AmbH : PMIOPort  Port=2  Side=Right  ConnectionType=Connection: foundation.thermal.thermal
  - : PMIOPort  Port=3  Side=Right
  iCell : Outport
  socCell : Outport  Port=2
  vCell : Outport  Port=3
  sohCell : Outport  Port=4
  tCell : Outport  Port=5
  wires:
  Balancing Command/1 -> Demux/1
  PS-Simulink Converter2/1 -> [socCell1]
  PS-Simulink Converter5/1 -> [socCell2]
  Demux/2 -> [BalancingComand2]
  PS-Simulink Converter/1 -> [iCell1]
  PS-Simulink Converter3/1 -> [iCell2]
  iCellMux/1 -> iCell/1
  vCellMux/1 -> vCell/1
  PS-Simulink Converter4/1 -> [vCell2]
  PS-Simulink Converter1/1 -> [vCell1]
  [BalancingComand2] -> Simulink-PS Converter1/1
  [BalancingComand1] -> Simulink-PS Converter/1
  socCellMux/1 -> socCell/1
  Demux/1 -> [BalancingComand1]
  PS-Simulink Converter7/1 -> Demux2/1
  Demux1/2 -> [sohCell1]
  sohCellMux/1 -> sohCell/1
  PS-Simulink Converter6/1 -> Demux1/1
  Demux2/2 -> [sohCell2]
  [socCell2] -> To Workspace14/1, socCellMux/2
  [socCell1] -> To Workspace13/1, socCellMux/1
  [sohCell1] -> To Workspace23/1, sohCellMux/1
  [sohCell2] -> To Workspace24/1, sohCellMux/2
  Probe1/1 -> To Workspace1/1, iCellMux1/2
  Probe/1 -> To Workspace2/1, iCellMux1/1
  iCellMux1/1 -> tCell/1
  Moving Average6/1(Out1) -> To Workspace16/1  "Average (500) V"
  Moving Average7/1(Out1) -> To Workspace17/1  "Average (500) V"
  Moving Average5/1(Out1) -> To Workspace6/1  "Average (500) i"
  Moving Average4/1(Out1) -> To Workspace5/1  "Average (500) i"
  [iCell1] -> Sensors - dSpace/1(Real Current1)
  [iCell2] -> Sensors - dSpace/2(Real Current2)
  Sensors - dSpace/1(Measured Current1) -> Moving Average4/1(Measured Current), To Workspace3/1, iCellMux/1  "i1"
  Sensors - dSpace/2(Measured Current2) -> Moving Average5/1(Measured Voltage), To Workspace4/1, iCellMux/2  "i2"
  [vCell1] -> Sensors - dSpace1/1(Real Voltage1)
  [vCell2] -> Sensors - dSpace1/2(Real Voltage2)
  Sensors - dSpace1/1(Measured Voltage1) -> Moving Average6/1(Measured Current), To Workspace19/1, vCellMux/1  "V1"
  Sensors - dSpace1/2(Measured Voltage2) -> Moving Average7/1(Measured Voltage), To Workspace18/1, vCellMux/2  "V2"
  connections:
  AmbH/RConn1 -- AmbH_From_1/LConn1 -- AmbH_From_2/LConn1
  Current Sensor1/LConn1 -- Resistor1/LConn1 -- +/RConn1 -- Resistor/LConn1 -- Current Sensor/LConn1
  TSPMeA-4/LConn2 -- Voltage Sensor1/LConn1 -- Current Sensor1/RConn2
  Voltage Sensor/RConn2 -- TSPMeA-3/RConn5 -- S1/RConn2 -- S2/RConn2 -- TSPMeA-4/RConn5 -- Voltage Sensor1/RConn2 -- -/RConn1
  Voltage Sensor/LConn1 -- TSPMeA-3/LConn2 -- Current Sensor/RConn2
  Current Sensor1/RConn1 -- PS-Simulink Converter3/LConn1
  Simulink-PS Converter/RConn1 -- S1/RConn1
  D1/LConn1 -- Resistor/RConn1
  TSPMeA-4/LConn1 -- AmbH_To_2/LConn1
  PS-Simulink Converter4/LConn1 -- Voltage Sensor1/RConn1
  S1/LConn1 -- D1/RConn1
  Current Sensor/RConn1 -- PS-Simulink Converter/LConn1
  PS-Simulink Converter5/LConn1 -- TSPMeA-4/RConn1
  PS-Simulink Converter2/LConn1 -- TSPMeA-3/RConn1
  D2/LConn1 -- Resistor1/RConn1
  S2/LConn1 -- D2/RConn1
  Simulink-PS Converter1/RConn1 -- S2/RConn1
  TSPMeA-3/LConn1 -- AmbH_To_1/LConn1
  Voltage Sensor/RConn1 -- PS-Simulink Converter1/LConn1
  TSPMeA-3/RConn3 -- PS-Simulink Converter6/LConn1
  TSPMeA-4/RConn3 -- PS-Simulink Converter7/LConn1
